simulink model "Question_4"  (R2024b)
settings: Solver=VariableStepAuto  StartTime=0.0  StopTime=10.0  RelTol=1e-3
model workspace (MAT data in the model file):
  B1 = 350
  B2 = 15020
  F = 100
  K1 = 80000
  K2 = 500000
  Mt = 2000
  Mv = 25000
settings Model: Creator=Sagar  LastModifiedBy=Sagar

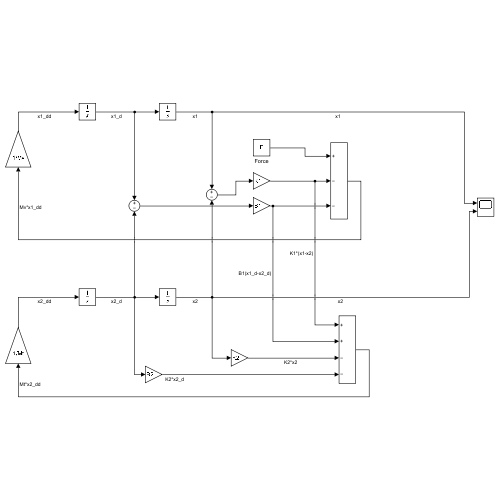
[thumbnail: Simulink's stored preview of the top-level diagram]
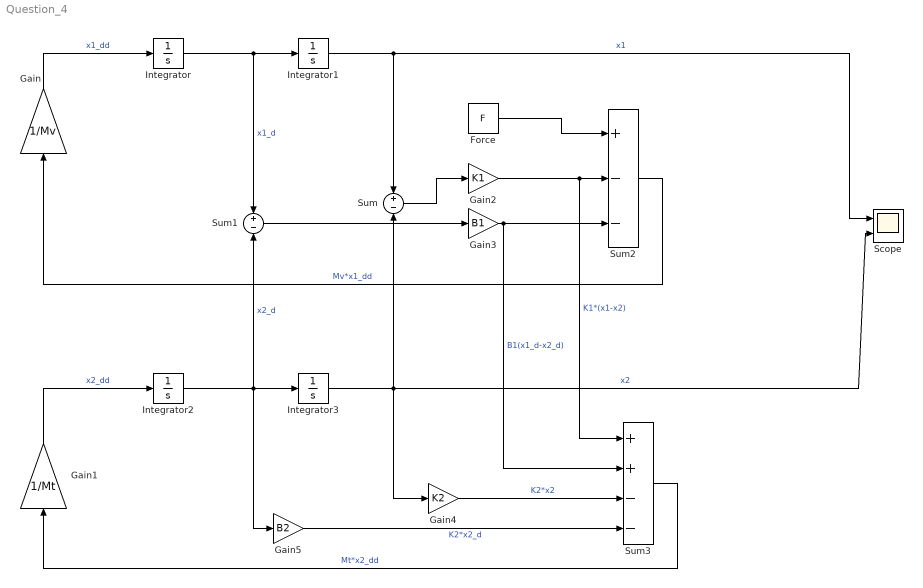
== system Question_4 ==
  Force : Constant  Value=F
  Gain : Gain  Gain=1/Mv
  Gain1 : Gain  Gain=1/Mt
  Gain2 : Gain  Gain=K1
  Gain3 : Gain  Gain=B1
  Gain4 : Gain  Gain=K2
  Gain5 : Gain  Gain=B2
  Integrator{,1..3} (4 alike) : Integrator
  Scope : Scope  NumInputPorts=2
  Sum : Sum  Inputs=+-
  Sum1 : Sum  Inputs=+-
  Sum2 : Sum  Inputs=+--
  Sum3 : Sum  Inputs=++--
  wires:
  Integrator/1 -> Sum1/1, Integrator1/1  "x1_d"
  Gain/1 -> Integrator/1  "x1_dd"
  Integrator1/1 -> Sum/1, Scope/1  "x1"
  Sum2/1 -> Gain/1  "Mv*x1_dd"
  Integrator3/1 -> Sum/2, Scope/2, Gain4/1  "x2"
  Gain1/1 -> Integrator2/1  "x2_dd"
  Integrator2/1 -> Sum1/2, Integrator3/1, Gain5/1  "x2_d"
  Sum3/1 -> Gain1/1  "Mt*x2_dd"
  Sum/1 -> Gain2/1
  Sum1/1 -> Gain3/1
  Gain2/1 -> Sum3/1, Sum2/2  "K1*(x1-x2)"
  Gain3/1 -> Sum3/2, Sum2/3  "B1(x1_d-x2_d)"
  Force/1 -> Sum2/1
  Gain4/1 -> Sum3/3  "K2*x2"
  Gain5/1 -> Sum3/4  "K2*x2_d"
